simulink model "Task20"  (R2022b)
settings: Solver=VariableStepAuto  StartTime=0.0  StopTime=10.0  RelTol=1e-3
settings Model: Creator=LOQ  LastModifiedBy=LOQ
settings OptimizationCC: ReuseModelBlockBuffer=on
settings RTWCC: GPUComputeCapability=5.0
settings ConfigComp: CovBoundaryAbsTol=1.0e-5

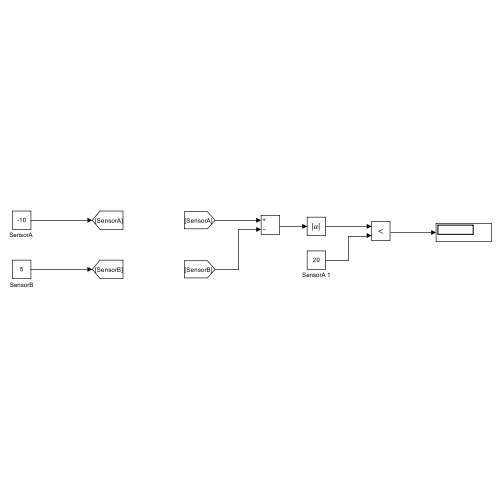
[thumbnail: Simulink's stored preview of the top-level diagram]
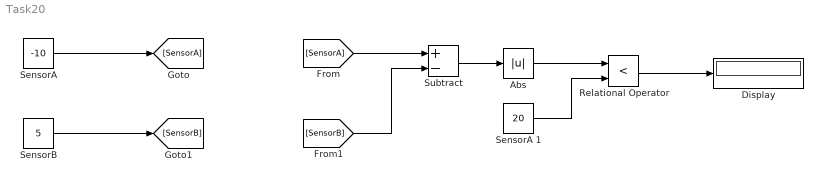
== system Task20 ==
  Abs : Abs  SaturateOnIntegerOverflow=off
  Display : Display
  Relational Operator : RelationalOperator  Operator=<  OutDataTypeStr=boolean  RndMeth=Simplest  InputSameDT=off
  "SensorA " : Constant  Value=-10
  SensorA 1 : Constant  Value=20
  SensorB : Constant  Value=5
  Subtract : Sum  Inputs=+-
  wires:
  "SensorA "/1 -> [SensorA]
  SensorB/1 -> [SensorB]
  [SensorA] -> Subtract/1
  [SensorB] -> Subtract/2
  Subtract/1 -> Abs/1
  Abs/1 -> Relational Operator/1
  SensorA 1/1 -> Relational Operator/2
  Relational Operator/1 -> Display/1
